simulink model "test_vacc_pkt_10_1_old"  (Simulink 7.2)
settings: Solver=ode45  StartTime=0.0  StopTime=5000  RelTol=1e-3
libraries: xbsIndex_r4 x248, xps_library x17, xbsReplacements_r4 x12, casper_library x5, casper_library_misc x2, casper_library_accumulators x1
(part 1 of 3)
settings Model: Creator=Jason Manley  LastModifiedBy=root
settings OptimizationCC: InitFltsAndDblsToZero=on
settings DebuggingCC: SaveWithParameterizedLinksMsg=none  SignalResolutionControl=TryResolveAllWithWarning  MultiTaskDSMMsg=warning  MultiTaskCondExecSysMsg=none  StrictBusMsg=None
settings RTWCC: IncludeERTFirstTime=on
settings GRTTargetCC: TargetFcnLib=ansi_tfl_tmw.mat

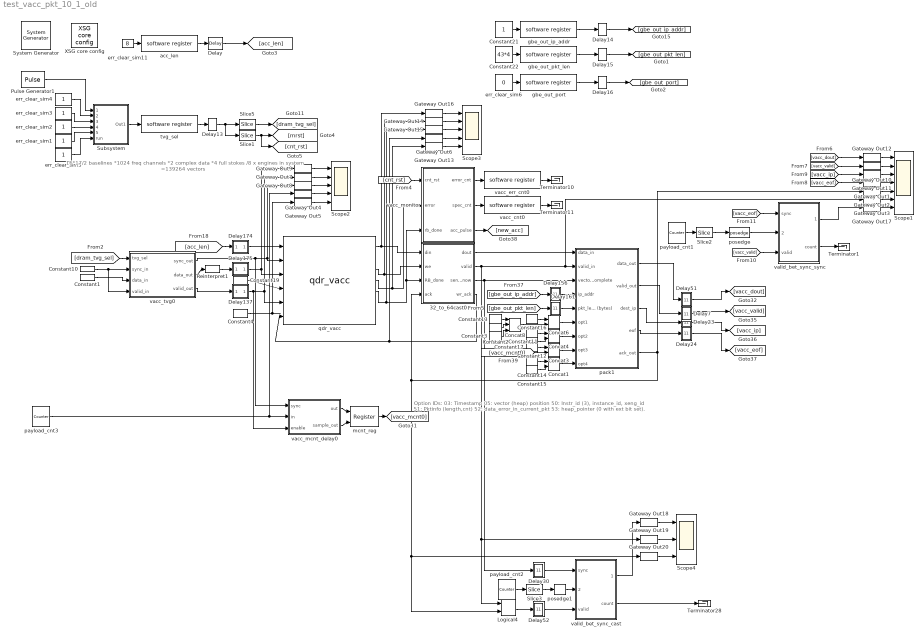
== system test_vacc_pkt_10_1_old ==
  note: 16*17/2 baselines
      | *1024 freq channels
      | *2 complex data
      | *4 full stokes
      | /8 x engines in system
      | =139264 vectors
  note: Option IDs:
      | 03: Timestamp
      | 05: vector (heap) position
      | 50: Instr_id (3), instance_id, xeng_id
      | 51: Pktinfo (length,cnt)
      | 52: data_error_in_current_pkt
      | 53: heap_pointer (0 with ext bit set).
  " System Generator" : xbsIndex_r4/ System Generator  Tag=genX  SystemSampleTime=-1  xilinxfamily=virtex5  part=xc5vlx110t  speed=-1  package=ff1136  synthesis_tool=XST  clock_wrapper=Clock Enables  directory=./test_vacc_pkt_10_1/sysgen  testbench=off  simulink_period=1  sysclk_period=5  dcm_input_clock_period=100  incr_netlist=off  trim_vbits=Everywhere in SubSystem  dbl_ovrd=According to Block Masks  core_generation=According to Block Masks  run_coregen=off  deprecated_control=off  eval_field=0  block_type=sysgen
      settings: block_version=10.1.3
  32_to_64cast0 : Subsystem
  Concat{1,3..4,6} (4 alike) : xbsIndex_r4/Concat  num_inputs=2  dbl_ovrd=off  block_type=concat
      settings: block_version=10.1.3
  Concat8 : xbsIndex_r4/Concat  num_inputs=3  dbl_ovrd=off  block_type=concat
      settings: block_version=10.1.3
  Constant1 : xbsIndex_r4/Constant  arith_type=Unsigned  const=0  n_bits=32  bin_pt=0  explicit_period=on  period=1  equ=P=C  opselect=C  inp2=PCIN>>17  opr=+  inp1=P  carry=CIN  dbl_ovrd=off  block_type=constant
  Constant10 : xbsIndex_r4/Constant  arith_type=Boolean  const=0  n_bits=1  bin_pt=0  explicit_period=on  period=1  equ=P=C  opselect=C  inp2=PCIN>>17  opr=+  inp1=P  carry=CIN  dbl_ovrd=off  block_type=constant
  Constant11 : xbsIndex_r4/Constant  arith_type=Unsigned  const=52  n_bits=16  bin_pt=0  explicit_period=on  period=1  equ=P=C  opselect=C  inp2=PCIN>>17  opr=+  inp1=P  carry=CIN  dbl_ovrd=off  block_type=constant
  Constant12 : xbsIndex_r4/Constant  arith_type=Unsigned  const=0  n_bits=48  bin_pt=0  explicit_period=on  period=1  equ=P=C  opselect=C  inp2=PCIN>>17  opr=+  inp1=P  carry=CIN  dbl_ovrd=off  block_type=constant
  Constant{2..3,13,17} (4 alike) : xbsIndex_r4/Constant  arith_type=Unsigned  const=3  n_bits=16  bin_pt=0  explicit_period=on  period=1  equ=P=C  opselect=C  inp2=PCIN>>17  opr=+  inp1=P  carry=CIN  dbl_ovrd=off  block_type=constant
  Constant14 : xbsIndex_r4/Constant  arith_type=Unsigned  const=53 + (1 * (2^15))  n_bits=16  bin_pt=0  explicit_period=on  period=1  equ=P=C  opselect=C  inp2=PCIN>>17  opr=+  inp1=P  carry=CIN  dbl_ovrd=off  block_type=constant
  Constant15 : xbsIndex_r4/Constant  arith_type=Unsigned  const=0  n_bits=48  bin_pt=0  explicit_period=on  period=1  equ=P=C  opselect=C  inp2=PCIN>>17  opr=+  inp1=P  carry=CIN  dbl_ovrd=off  block_type=constant
  Constant16 : xbsIndex_r4/Constant  arith_type=Unsigned  const=50  n_bits=16  bin_pt=0  explicit_period=on  period=1  equ=P=C  opselect=C  inp2=PCIN>>17  opr=+  inp1=P  carry=CIN  dbl_ovrd=off  block_type=constant
  Constant19 : xbsIndex_r4/Constant  arith_type=Unsigned  const=0  n_bits=4  bin_pt=0  explicit_period=on  period=1  equ=P=C  opselect=C  inp2=PCIN>>17  opr=+  inp1=P  carry=CIN  dbl_ovrd=off  block_type=constant
  Constant21 : Constant  OutDataType=sfix(16)  OutScaling=2^0
  Constant22 : Constant  Value=43*4  OutDataType=sfix(16)  OutScaling=2^0
  Constant4 : xbsIndex_r4/Constant  arith_type=Unsigned  const=0  n_bits=4  bin_pt=0  explicit_period=on  period=1  equ=P=C  opselect=C  inp2=PCIN>>17  opr=+  inp1=P  carry=CIN  dbl_ovrd=off  block_type=constant
  Delay : xbsIndex_r4/Delay  en=off  latency=1  dbl_ovrd=off  reg_retiming=on  block_type=delay
  Delay{13..16} (4 alike) : xbsIndex_r4/Delay  en=off  latency=2  dbl_ovrd=off  reg_retiming=on  block_type=delay
      settings: xl_area=[0, 0, 0, 0, 0, 0, 0]
  Delay137 : Subsystem  AncestorBlock=casper_library/Delays/pipeline  mask(pipeline){latency=2}
      mask help:
      | An explicitly laid-out delay line to avoid mapping to SRL16s
      | for use in pipelining to help achieve timing closure.
      mask init:
      | pipeline_init(gcb, 'latency', latency);
      mask Display:
      | port_label('input', 1, 'd');
      | port_label('output', 1, 'q');
      | disp(['Z^-', num2str(latency)]);
  Delay156 : Subsystem  AncestorBlock=casper_library/Delays/pipeline  mask(pipeline){latency=5}
      mask help:
      | An explicitly laid-out delay line to avoid mapping to SRL16s
      | for use in pipelining to help achieve timing closure.
      mask init:
      | pipeline_init(gcb, 'latency', latency);
      mask Display:
      | port_label('input', 1, 'd');
      | port_label('output', 1, 'q');
      | disp(['Z^-', num2str(latency)]);
  Delay161 : Subsystem  AncestorBlock=casper_library/Delays/pipeline  mask(pipeline){latency=1}
      mask help:
      | An explicitly laid-out delay line to avoid mapping to SRL16s
      | for use in pipelining to help achieve timing closure.
      mask init:
      | pipeline_init(gcb, 'latency', latency);
      mask Display:
      | port_label('input', 1, 'd');
      | port_label('output', 1, 'q');
      | disp(['Z^-', num2str(latency)]);
  Delay174 : Subsystem  AncestorBlock=casper_library/Delays/pipeline  mask(pipeline){latency=2}
      mask help:
      | An explicitly laid-out delay line to avoid mapping to SRL16s
      | for use in pipelining to help achieve timing closure.
      mask init:
      | pipeline_init(gcb, 'latency', latency);
      mask Display:
      | port_label('input', 1, 'd');
      | port_label('output', 1, 'q');
      | disp(['Z^-', num2str(latency)]);
  Delay175 : Subsystem  AncestorBlock=casper_library/Delays/pipeline  mask(pipeline){latency=2}
      mask help:
      | An explicitly laid-out delay line to avoid mapping to SRL16s
      | for use in pipelining to help achieve timing closure.
      mask init:
      | pipeline_init(gcb, 'latency', latency);
      mask Display:
      | port_label('input', 1, 'd');
      | port_label('output', 1, 'q');
      | disp(['Z^-', num2str(latency)]);
  Delay23 : Subsystem  AncestorBlock=casper_library/Delays/pipeline  mask(pipeline){latency=2}
      mask help:
      | An explicitly laid-out delay line to avoid mapping to SRL16s
      | for use in pipelining to help achieve timing closure.
      mask init:
      | pipeline_init(gcb, 'latency', latency);
      mask Display:
      | port_label('input', 1, 'd');
      | port_label('output', 1, 'q');
      | disp(['Z^-', num2str(latency)]);
  Delay24 : Subsystem  AncestorBlock=casper_library/Delays/pipeline  mask(pipeline){latency=2}
      mask help:
      | An explicitly laid-out delay line to avoid mapping to SRL16s
      | for use in pipelining to help achieve timing closure.
      mask init:
      | pipeline_init(gcb, 'latency', latency);
      mask Display:
      | port_label('input', 1, 'd');
      | port_label('output', 1, 'q');
      | disp(['Z^-', num2str(latency)]);
  Delay30 : Subsystem  AncestorBlock=casper_library/Delays/pipeline  mask(pipeline){latency=2}
      mask help:
      | An explicitly laid-out delay line to avoid mapping to SRL16s
      | for use in pipelining to help achieve timing closure.
      mask init:
      | pipeline_init(gcb, 'latency', latency);
      mask Display:
      | port_label('input', 1, 'd');
      | port_label('output', 1, 'q');
      | disp(['Z^-', num2str(latency)]);
  Delay51 : Subsystem  AncestorBlock=casper_library/Delays/pipeline  mask(pipeline){latency=2}
      mask help:
      | An explicitly laid-out delay line to avoid mapping to SRL16s
      | for use in pipelining to help achieve timing closure.
      mask init:
      | pipeline_init(gcb, 'latency', latency);
      mask Display:
      | port_label('input', 1, 'd');
      | port_label('output', 1, 'q');
      | disp(['Z^-', num2str(latency)]);
  Delay52 : Subsystem  AncestorBlock=casper_library/Delays/pipeline  mask(pipeline){latency=2}
      mask help:
      | An explicitly laid-out delay line to avoid mapping to SRL16s
      | for use in pipelining to help achieve timing closure.
      mask init:
      | pipeline_init(gcb, 'latency', latency);
      mask Display:
      | port_label('input', 1, 'd');
      | port_label('output', 1, 'q');
      | disp(['Z^-', num2str(latency)]);
  Delay7 : Subsystem  AncestorBlock=casper_library/Delays/pipeline  mask(pipeline){latency=2}
      mask help:
      | An explicitly laid-out delay line to avoid mapping to SRL16s
      | for use in pipelining to help achieve timing closure.
      mask init:
      | pipeline_init(gcb, 'latency', latency);
      mask Display:
      | port_label('input', 1, 'd');
      | port_label('output', 1, 'q');
      | disp(['Z^-', num2str(latency)]);
  Gateway Out{1..20} (20 alike) : xbsIndex_r4/Gateway Out  hdl_port=off  timing_constraint=None  locs_specified=off  LOCs={}  block_type=gatewayout
      settings: infoedit="Gateway out block.  Converts Xilinx fixed point inputs into ouputs of type Simulink integer, double, or fixed point.<P><P>Hardware notes:  In hardware these blocks become top level output ports or are discarded, depending on how they are configured."  xl_area=[0, 0, 0, 0, 0, 0, 0]  block_version=10.1.3
  Logical4 : xbsIndex_r4/Logical  logical_function=AND  inputs=2  en=off  latency=1  precision=Full  arith_type=Unsigned  n_bits=8  bin_pt=2  align_bp=on  dbl_ovrd=off  block_type=logical
      settings: xl_area=[0, 0, 0, 0, 0, 0, 0]
  Pulse Generator1 : DiscretePulseGenerator  Period=2*100*8  PhaseDelay=3
  Reinterpret1 : xbsIndex_r4/Reinterpret  force_arith_type=on  arith_type="Signed  (2's comp)"  force_bin_pt=on  bin_pt=0  block_type=reinterpret
      settings: infoedit="Changes signal type without altering the binary representation.   You can changed the signal between signed and unsigned, and relocate the binary point.<P><P>Hardware notes: In hardware this block costs nothing.<P><P>Example:  Suppose the input is 6 bits wide, signed, with 2 fractional bits, and the output is forced to unsigned with 0 fractional bits.  Then an input of -2.0 (1110.00 in binary 2's complement) becomes an output of 56 (111000 in binary)."  block_version=10.1.3
  Scope1 : Scope  NumInputPorts=7
      settings: YMin=0~0~0.95~0~0~0~493.05  YMax=1e+019~1~1.05~1~1~1~544.95  SaveName=ScopeData7
  Scope2 : Scope  NumInputPorts=5
      settings: YMin=0.95~0~-1~-5~-5  YMax=1.05~1~1~5~5  SaveName=ScopeData8
  Scope3 : Scope  NumInputPorts=5
      settings: YMin=0.95~0~-1~-5~-5  YMax=1.05~1~1~5~5  SaveName=ScopeData10
  Scope4 : Scope  NumInputPorts=3
      settings: YMin=61000~0~0  YMax=69500~1~1  SaveName=ScopeData11
  Slice1 : xbsIndex_r4/Slice  nbits=1  boolean_output=on  mode=Lower Bit Location + Width  bit1=0  base1=MSB of Input  bit0=31  base0=LSB of Input  dbl_ovrd=off  block_type=slice
      settings: infoedit="Extracts a given range of bits from each input sample and presents it at the output.  The output type is ordinarily unsigned with binary point at zero, but can be Boolean when the slice is one bit wide.<P><P>Hardware notes: In hardware this block costs nothing."  block_version=10.1.3
  Slice2 : xbsIndex_r4/Slice  nbits=1  boolean_output=on  mode=Upper Bit Location + Width  bit1=0  base1=MSB of Input  bit0=1  base0=LSB of Input  dbl_ovrd=off  block_type=slice
      settings: infoedit="Extracts a given range of bits from each input sample and presents it at the output.  The output type is ordinarily unsigned with binary point at zero, but can be Boolean when the slice is one bit wide.<P><P>Hardware notes: In hardware this block costs nothing."  block_version=10.1.3
  Slice3 : xbsIndex_r4/Slice  nbits=1  boolean_output=on  mode=Upper Bit Location + Width  bit1=0  base1=MSB of Input  bit0=1  base0=LSB of Input  dbl_ovrd=off  block_type=slice
      settings: infoedit="Extracts a given range of bits from each input sample and presents it at the output.  The output type is ordinarily unsigned with binary point at zero, but can be Boolean when the slice is one bit wide.<P><P>Hardware notes: In hardware this block costs nothing."  block_version=10.1.3
  Slice5 : xbsIndex_r4/Slice  nbits=6  boolean_output=off  mode=Lower Bit Location + Width  bit1=0  base1=MSB of Input  bit0=9  base0=LSB of Input  dbl_ovrd=off  block_type=slice
      settings: infoedit="Extracts a given range of bits from each input sample and presents it at the output.  The output type is ordinarily unsigned with binary point at zero, but can be Boolean when the slice is one bit wide.<P><P>Hardware notes: In hardware this block costs nothing."  block_version=10.1.3
  Subsystem : Subsystem
  Terminator{1,10..11,28} (4 alike) : Terminator
  XSG core config : xps_library/XSG core config  Tag=xps:xsg  SystemSampleTime=-1  hw_sys=iBOB  ibob_linux=off  clk_src=sys_clk  iBOB_clk_src=sys_clk  BEE2_ctrl_clk_src=sys_clk  BEE2_usr_clk_src=sys_clk  ROACH_clk_src=arb_clk  CORR_clk_src=sys_clk  gpio_clk_io_group=iBOB:sma  gpio_clk_bit_index=0  clk_rate=100  sample_period=1  synthesis_tool=XST  mpc_type=powerpc405
  acc_len : xps_library/software register  Tag=xps:sw_reg  SystemSampleTime=-1  io_dir=From Processor  arith_type=Unsigned  bitwidth=32  bin_pt=0  sample_period=1  gw_name=test_vacc_pkt_10_1_acc_len_user_data_out
      link override qdr_vacc_tvg_sel_user_data_out: arith_type=Unsigned  n_bits=32  bin_pt=0  period=1
      link override test_d_v_p_10_1_new_packet_format_acc_len_user_data_out: arith_type=Unsigned  n_bits=32  bin_pt=0  period=1
      link override test_qdr_vacc_acc_len_user_data_out: arith_type=Unsigned  n_bits=32  bin_pt=0  period=1
      link override test_qdr_vacc_tvg_sel_user_data_out: arith_type=Unsigned  n_bits=32  bin_pt=0  period=1
      link override test_vacc_10_1_new_pkt_form_acc_len_user_data_out: arith_type=Unsigned  n_bits=32  bin_pt=0  period=1
      link override test_vacc_pkt_10_1_acc_len_user_data_out: arith_type=Unsigned  n_bits=32  bin_pt=0  period=1
  err_clear_sim{1..5} (5 alike) : Constant  OutDataType=sfix(16)  OutScaling=2^0
  err_clear_sim11 : Constant  Value=8  OutDataType=sfix(16)  OutScaling=2^0
  err_clear_sim6 : Constant  Value=0  OutDataType=sfix(16)  OutScaling=2^0
  gbe_out_ip_addr : xps_library/software register  Tag=xps:sw_reg  SystemSampleTime=-1  io_dir=From Processor  arith_type=Unsigned  bitwidth=32  bin_pt=0  sample_period=1  gw_name=test_vacc_pkt_10_1_gbe_out_ip_addr_user_data_out
      link override test_d_v_p_10_1_new_packet_format_gbe_out_ip_addr_user_data_out: arith_type=Unsigned  n_bits=32  bin_pt=0  period=1
      link override test_d_v_p_10_1_new_packet_format_out_ip_addr_user_data_out: arith_type=Unsigned  n_bits=32  bin_pt=0  period=1
      link override test_vacc_10_1_new_pkt_form_gbe_out_ip_addr_user_data_out: arith_type=Unsigned  n_bits=32  bin_pt=0  period=1
      link override test_vacc_pkt_10_1_gbe_out_ip_addr_user_data_out: arith_type=Unsigned  n_bits=32  bin_pt=0  period=1
  gbe_out_pkt_len : xps_library/software register  Tag=xps:sw_reg  SystemSampleTime=-1  io_dir=From Processor  arith_type=Unsigned  bitwidth=32  bin_pt=0  sample_period=1  gw_name=test_vacc_pkt_10_1_gbe_out_pkt_len_user_data_out
      link override test_d_v_p_10_1_new_packet_format_gbe_out_pkt_len_user_data_out: arith_type=Unsigned  n_bits=32  bin_pt=0  period=1
      link override test_d_v_p_10_1_new_packet_format_pkt_len_user_data_out: arith_type=Unsigned  n_bits=32  bin_pt=0  period=1
      link override test_vacc_10_1_new_pkt_form_gbe_out_pkt_len_user_data_out: arith_type=Unsigned  n_bits=32  bin_pt=0  period=1
      link override test_vacc_pkt_10_1_gbe_out_pkt_len_user_data_out: arith_type=Unsigned  n_bits=32  bin_pt=0  period=1
  gbe_out_port : xps_library/software register  Tag=xps:sw_reg  SystemSampleTime=-1  io_dir=From Processor  arith_type=Unsigned  bitwidth=32  bin_pt=0  sample_period=1  gw_name=test_vacc_pkt_10_1_gbe_out_port_user_data_out
      link override test_d_v_p_10_1_new_packet_format_gbe_out_port_user_data_out: arith_type=Unsigned  n_bits=32  bin_pt=0  period=1
      link override test_vacc_10_1_new_pkt_form_gbe_out_port_user_data_out: arith_type=Unsigned  n_bits=32  bin_pt=0  period=1
      link override test_vacc_pkt_10_1_gbe_out_port_user_data_out: arith_type=Unsigned  n_bits=32  bin_pt=0  period=1
  mcnt_reg : xbsIndex_r4/Register  init=0  rst=off  en=on  dbl_ovrd=off  block_type=register
  pack1 : Subsystem  mask(pkt_pack_mask){vector_len=100, magic_id=hex2dec('4b52'), ver_id=3}
      mask prompts: vector_len "vector length"; magic_id "Magic Identifier"; ver_id "Version Identifier"
      mask help:
      | This block generates packets from a datastream.
      |
      | Packets are created with a fixed header followed by a user-specified number of 64-bit options.
      |
      | Requires a 64-bit data stream.
      |
      | See the documentation for further details.
      mask init:
      | vector_bits = ceil(log2(vector_len));
  payload_cnt1 : xbsIndex_r4/Counter  cnt_type=Free Running  cnt_to=0  operation=Up  start_count=0  cnt_by_val=1  arith_type=Unsigned  n_bits=12  bin_pt=0  load_pin=off  rst=off  en=off  explicit_period=on  period=1  dbl_ovrd=off  use_behavioral_HDL=off  implementation=Fabric  use_rpm=on  block_type=counter
      settings: xl_area=[0, 0, 0, 0, 0, 0, 0]
  payload_cnt2 : xbsIndex_r4/Counter  cnt_type=Free Running  cnt_to=0  operation=Up  start_count=0  cnt_by_val=1  arith_type=Unsigned  n_bits=19  bin_pt=0  load_pin=off  rst=off  en=off  explicit_period=on  period=1  dbl_ovrd=off  use_behavioral_HDL=off  implementation=Fabric  use_rpm=on  block_type=counter
      settings: xl_area=[0, 0, 0, 0, 0, 0, 0]
  payload_cnt3 : xbsIndex_r4/Counter  cnt_type=Free Running  cnt_to=0  operation=Up  start_count=0  cnt_by_val=1  arith_type=Unsigned  n_bits=48  bin_pt=0  load_pin=off  rst=off  en=off  explicit_period=on  period=1  dbl_ovrd=off  use_behavioral_HDL=off  implementation=Fabric  use_rpm=on  block_type=counter
      settings: xl_area=[0, 0, 0, 0, 0, 0, 0]
  posedge : casper_library_misc/posedge  Tag=Rising Edge Detector  SystemSampleTime=-1
  posedge1 : casper_library_misc/posedge  Tag=Rising Edge Detector  SystemSampleTime=-1
  qdr_vacc : casper_library_accumulators/qdr_vacc  SystemSampleTime=-1  vector_len=100
      settings: AttributesFormatString=Vector Length: 100
  tvg_sel : xps_library/software register  Tag=xps:sw_reg  SystemSampleTime=-1  io_dir=From Processor  arith_type=Unsigned  bitwidth=32  bin_pt=0  sample_period=1  gw_name=test_vacc_pkt_10_1_tvg_sel_user_data_out
      link override test_d_v_p_10_1_new_packet_format_tvg_sel_user_data_out: arith_type=Unsigned  n_bits=32  bin_pt=0  period=1
      link override test_vacc_10_1_new_pkt_form_tvg_sel_user_data_out: arith_type=Unsigned  n_bits=32  bin_pt=0  period=1
      link override test_vacc_pkt_10_1_tvg_sel_user_data_out: arith_type=Unsigned  n_bits=32  bin_pt=0  period=1
  vacc_cnt0 : xps_library/software register  Tag=xps:sw_reg  SystemSampleTime=-1  io_dir=To Processor  arith_type=Unsigned  bitwidth=32  bin_pt=0  sample_period=1  gw_name=test_vacc_pkt_10_1_vacc_cnt0_user_data_in
      link override convert: arith_type=Unsigned  n_bits=32  bin_pt=0
  vacc_err_cnt0 : xps_library/software register  Tag=xps:sw_reg  SystemSampleTime=-1  io_dir=To Processor  arith_type=Unsigned  bitwidth=32  bin_pt=0  sample_period=1  gw_name=test_vacc_pkt_10_1_vacc_err_cnt0_user_data_in
      link override convert: arith_type=Unsigned  n_bits=32  bin_pt=0
  vacc_mcnt_delay0 : Subsystem  mask(sample_and_hold){period=16*17/2*1024*2*4/8}
      mask prompts: period "Sample period (clocks)"
      mask help: This block will sample an input signal at a user specified rate and hold the value on the output.
  vacc_monitor : Subsystem
  vacc_tvg0 : Subsystem  AncestorBlock=casper_library/Accumulators/vacc_tvg  mask{len=100}
      mask prompts: len "Number of Vectors"
      mask init:
      | fmtstr = sprintf('Vector Length: %d', len);
      | set_param(gcb, 'AttributesFormatString', fmtstr);
      settings: AttributesFormatString=Vector Length: 100
  valid_bet_sync_cast : Subsystem
  valid_bet_sync_sync : Subsystem
  wires:
  tvg_sel/1 -> Delay13/1
  Slice5/1 -> [dram_tvg_sel]
  err_clear_sim1/1 -> Subsystem/5(data_sel)
  err_clear_sim2/1 -> Subsystem/4(valid_sel)
  err_clear_sim3/1 -> Subsystem/3(inj_vector)
  err_clear_sim4/1 -> Subsystem/2(inj_counter)
  Subsystem/1(Out1) -> tvg_sel/1
  Pulse Generator1/1 -> Subsystem/1(new_acc)
  err_clear_sim5/1 -> Subsystem/6(run)
  Constant22/1 -> gbe_out_pkt_len/1
  Constant21/1 -> gbe_out_ip_addr/1
  gbe_out_ip_addr/1 -> Delay14/1
  gbe_out_pkt_len/1 -> Delay15/1
  Slice1/1 -> [mrst], [cnt_rst]
  acc_len/1 -> Delay/1
  err_clear_sim11/1 -> acc_len/1
  err_clear_sim6/1 -> gbe_out_port/1
  gbe_out_port/1 -> Delay16/1
  Delay13/1 -> Slice5/1, Slice1/1
  Delay14/1 -> [gbe_out_ip_addr]
  Delay15/1 -> [gbe_out_pkt_len]
  Delay16/1 -> [gbe_out_port]
  qdr_vacc/1 -> 32_to_64cast0/1(din), Gateway Out16/1
  qdr_vacc/3 -> 32_to_64cast0/2(we), Gateway Out14/1
  qdr_vacc/5 -> 32_to_64cast0/3(RB_done), vacc_monitor/3(rb_done), Gateway Out15/1
  [acc_len] -> Delay174/1(d)
  Delay174/1(q) -> qdr_vacc/1
  Delay175/1(q) -> Gateway Out9/1, qdr_vacc/3
  Delay137/1(q) -> vacc_mcnt_delay0/3(enable), Gateway Out7/1, qdr_vacc/5
  [gbe_out_ip_addr] -> Delay156/1(d)
  [gbe_out_pkt_len] -> Delay161/1(d)
  Delay156/1(q) -> pack1/4(ip_addr)
  Delay161/1(q) -> pack1/5(pkt_len (bytes))
  pack1/4(eof) -> Delay24/1(d)
  pack1/5(ack_out) -> Gateway Out2/1, 32_to_64cast0/4(ack), Logical4/2, Gateway Out20/1
  pack1/1(data_out) -> Delay51/1(d)
  pack1/2(valid_out) -> Delay7/1(d)
  32_to_64cast0/1(dout) -> pack1/1(data_in)
  32_to_64cast0/2(valid) -> pack1/2(valid_in), Gateway Out3/1, Logical4/1, Gateway Out19/1
  32_to_64cast0/3(send_now) -> pack1/3(vector_complete), Delay30/1(d)
  32_to_64cast0/4(wr_ack) -> Gateway Out6/1, qdr_vacc/6
  pack1/3(dest_ip) -> Delay23/1(d)
  Constant4/1 -> Gateway Out5/1
  Constant19/1 -> qdr_vacc/4
  Delay51/1(q) -> [vacc_dout]
  Delay7/1(q) -> [vacc_valid]
  Delay23/1(q) -> [vacc_ip]
  Delay24/1(q) -> [vacc_eof]
  vacc_tvg0/1(sync_out) -> vacc_mcnt_delay0/1(sync), Gateway Out8/1, qdr_vacc/2
  vacc_tvg0/2(data_out) -> Reinterpret1/1
  vacc_tvg0/3(valid_out) -> Delay137/1(d)
  vacc_mcnt_delay0/1(out) -> mcnt_reg/1
  vacc_mcnt_delay0/2(sample_out) -> mcnt_reg/2
  Constant17/1 -> Concat3/1
  [vacc_mcnt0] -> Concat3/2
  mcnt_reg/1 -> [vacc_mcnt0]
  Concat3/1 -> pack1/8(opt3)
  Concat6/1 -> pack1/6(opt1)
  Constant16/1 -> Concat6/1
  Concat4/1 -> pack1/7(opt2)
  Concat1/1 -> pack1/9(opt4)
  vacc_cnt0/1 -> Terminator11/1
  vacc_monitor/2(spec_cnt) -> vacc_cnt0/1
  Reinterpret1/1 -> Delay175/1(d)
  vacc_err_cnt0/1 -> Terminator10/1
  vacc_monitor/1(error_cnt) -> vacc_err_cnt0/1
  qdr_vacc/4 -> vacc_monitor/2(error), Gateway Out13/1
  vacc_monitor/3(acc_pulse) -> [new_acc]
  [cnt_rst] -> vacc_monitor/1(cnt_rst)
  Concat8/1 -> Concat6/2
  Constant13/1 -> Concat8/1
  Constant2/1 -> Concat8/2
  Constant3/1 -> Concat8/3
  Constant14/1 -> Concat1/1
  Constant15/1 -> Concat1/2
  Constant11/1 -> Concat4/1
  Constant12/1 -> Concat4/2
  Delay/1 -> [acc_len]
  [dram_tvg_sel] -> vacc_tvg0/1(tvg_sel)
  Constant10/1 -> vacc_tvg0/2(sync_in), vacc_tvg0/4(valid_in)
  Constant1/1 -> vacc_tvg0/3(data_in)
  payload_cnt3/1 -> vacc_mcnt_delay0/2(in), Gateway Out4/1
  Gateway Out5/1 -> Scope2/5
  Gateway Out4/1 -> Scope2/4
  Gateway Out9/1 -> Scope2/1
  Gateway Out7/1 -> Scope2/2
  Gateway Out8/1 -> Scope2/3
  Gateway Out3/1 -> Scope1/6
  Gateway Out2/1 -> Scope1/5
  Gateway Out1/1 -> Scope1/4
  Gateway Out12/1 -> Scope1/1
  Gateway Out10/1 -> Scope1/2
  Gateway Out11/1 -> Scope1/3
  [vacc_dout] -> Gateway Out12/1
  [vacc_valid] -> Gateway Out10/1
  [vacc_ip] -> Gateway Out11/1
  [vacc_eof] -> Gateway Out1/1
  Gateway Out13/1 -> Scope3/5
  Gateway Out6/1 -> Scope3/4
  Gateway Out16/1 -> Scope3/1
  Gateway Out14/1 -> Scope3/2
  Gateway Out15/1 -> Scope3/3
  valid_bet_sync_sync/2(count) -> Terminator1/1
  [vacc_valid] -> valid_bet_sync_sync/3(valid)
  [vacc_eof] -> valid_bet_sync_sync/1(sync)
  payload_cnt1/1 -> Slice2/1
  Slice2/1 -> posedge/1
  Gateway Out17/1 -> Scope1/7
  posedge/1 -> valid_bet_sync_sync/2(rst_max)
  Logical4/1 -> Delay52/1(d)
  valid_bet_sync_cast/2(count) -> Terminator28/1
  valid_bet_sync_cast/1(max_count) -> Gateway Out18/1
  Delay30/1(q) -> valid_bet_sync_cast/1(sync)
  Slice3/1 -> posedge1/1
  Delay52/1(q) -> valid_bet_sync_cast/3(valid)
  Gateway Out18/1 -> Scope4/1
  Gateway Out19/1 -> Scope4/2
  Gateway Out20/1 -> Scope4/3
  payload_cnt2/1 -> Slice3/1
  posedge1/1 -> valid_bet_sync_cast/2(rst_max)
  valid_bet_sync_sync/1(max_count) -> Gateway Out17/1

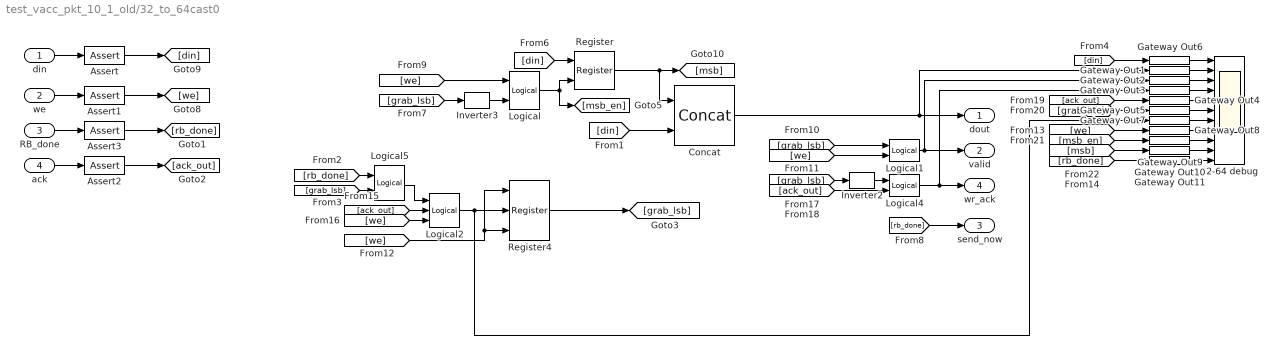
== system test_vacc_pkt_10_1_old/32_to_64cast0 ==
  din : Inport  OutDataType=sfix(16)  OutScaling=2^0
  we : Inport  Port=2  OutDataType=sfix(16)  OutScaling=2^0
  RB_done : Inport  Port=3  OutDataType=sfix(16)  OutScaling=2^0
  ack : Inport  Port=4  OutDataType=sfix(16)  OutScaling=2^0
  32-64 debug : Scope  NumInputPorts=11
      settings: YMin=-1~0~0~0~-5~-5~-5~-5~-5~-5~-5  YMax=1~150~1~1~5~5~5~5~5~5~5  SaveName=ScopeData5
  Assert : xbsIndex_r4/Assert  assert_type=on  type_source=Explicitly  arith_type=Unsigned  n_bits=32  bin_pt=0  assert_rate=off  rate_source=Explicitly  period=1  output_port=on  block_type=assert
      settings: infoedit=Asserts a user-defined sample rate and/or type on a signal.<P><P>Hardware notes: In hardware this block costs nothing.  block_version=10.1.3
  Assert1 : xbsIndex_r4/Assert  assert_type=on  type_source=Explicitly  arith_type=Boolean  n_bits=32  bin_pt=0  assert_rate=off  rate_source=Explicitly  period=1  output_port=on  block_type=assert
      settings: infoedit=Asserts a user-defined sample rate and/or type on a signal.<P><P>Hardware notes: In hardware this block costs nothing.  block_version=10.1.3
  Assert2 : xbsIndex_r4/Assert  assert_type=on  type_source=Explicitly  arith_type=Boolean  n_bits=32  bin_pt=0  assert_rate=off  rate_source=Explicitly  period=1  output_port=on  block_type=assert
      settings: infoedit=Asserts a user-defined sample rate and/or type on a signal.<P><P>Hardware notes: In hardware this block costs nothing.  block_version=10.1.3
  Assert3 : xbsIndex_r4/Assert  assert_type=on  type_source=Explicitly  arith_type=Boolean  n_bits=32  bin_pt=0  assert_rate=off  rate_source=Explicitly  period=1  output_port=on  block_type=assert
      settings: infoedit=Asserts a user-defined sample rate and/or type on a signal.<P><P>Hardware notes: In hardware this block costs nothing.  block_version=10.1.3
  Concat : xbsIndex_r4/Concat  num_inputs=2  dbl_ovrd=off  block_type=concat
      settings: block_version=10.1.3
  Gateway Out{1..11} (11 alike) : xbsIndex_r4/Gateway Out  hdl_port=off  timing_constraint=None  locs_specified=off  LOCs={}  block_type=gatewayout
      settings: infoedit="Gateway out block.  Converts Xilinx fixed point inputs into ouputs of type Simulink integer, double, or fixed point.<P><P>Hardware notes:  In hardware these blocks become top level output ports or are discarded, depending on how they are configured."  xl_area=[0, 0, 0, 0, 0, 0, 0]  block_version=10.1.3
  Inverter2 : xbsIndex_r4/Inverter  en=off  latency=0  dbl_ovrd=off  block_type=inv
  Inverter3 : xbsIndex_r4/Inverter  en=off  latency=0  dbl_ovrd=off  block_type=inv
  Logical : xbsIndex_r4/Logical  logical_function=AND  inputs=2  en=off  latency=0  precision=Full  arith_type=Unsigned  n_bits=16  bin_pt=0  align_bp=on  dbl_ovrd=off  block_type=logical
  Logical1 : xbsIndex_r4/Logical  logical_function=AND  inputs=2  en=off  latency=0  precision=Full  arith_type=Unsigned  n_bits=16  bin_pt=0  align_bp=on  dbl_ovrd=off  block_type=logical
  Logical2 : xbsIndex_r4/Logical  logical_function=AND  inputs=3  en=off  latency=0  precision=Full  arith_type=Unsigned  n_bits=16  bin_pt=0  align_bp=on  dbl_ovrd=off  block_type=logical
  Logical4 : xbsIndex_r4/Logical  logical_function=OR  inputs=2  en=off  latency=0  precision=Full  arith_type=Unsigned  n_bits=16  bin_pt=0  align_bp=on  dbl_ovrd=off  block_type=logical
  Logical5 : xbsIndex_r4/Logical  logical_function=OR  inputs=2  en=off  latency=0  precision=Full  arith_type=Unsigned  n_bits=16  bin_pt=0  align_bp=on  dbl_ovrd=off  block_type=logical
  Register : xbsIndex_r4/Register  init=0  rst=off  en=on  dbl_ovrd=off  block_type=register
  Register4 : xbsIndex_r4/Register  init=0  rst=on  en=on  dbl_ovrd=off  block_type=register
  dout : Outport  OutDataType=sfix(16)  OutScaling=2^0
  valid : Outport  Port=2  OutDataType=sfix(16)  OutScaling=2^0
  send_now : Outport  Port=3  OutDataType=sfix(16)  OutScaling=2^0
  wr_ack : Outport  Port=4  OutDataType=sfix(16)  OutScaling=2^0
  wires:
  din/1 -> Assert/1
  ack/1 -> Assert2/1
  we/1 -> Assert1/1
  Assert/1 -> [din]
  Assert1/1 -> [we]
  Assert2/1 -> [ack_out]
  [din] -> Register/1
  Register/1 -> Concat/1, [msb]
  [din] -> Concat/2
  Logical4/1 -> wr_ack/1, Gateway Out3/1
  Logical1/1 -> valid/1, Gateway Out2/1
  Logical/1 -> Register/2, [msb_en]
  RB_done/1 -> Assert3/1
  Assert3/1 -> [rb_done]
  [rb_done] -> send_now/1
  Concat/1 -> dout/1, Gateway Out1/1
  Register4/1 -> [grab_lsb]
  [grab_lsb] -> Inverter3/1
  [we] -> Logical/1
  [grab_lsb] -> Inverter2/1
  [ack_out] -> Logical4/2
  Gateway Out6/1 -> 32-64 debug/1
  Gateway Out1/1 -> 32-64 debug/2
  Gateway Out2/1 -> 32-64 debug/3
  Gateway Out3/1 -> 32-64 debug/4
  [din] -> Gateway Out6/1
  [ack_out] -> Gateway Out4/1
  [grab_lsb] -> Gateway Out5/1
  Gateway Out4/1 -> 32-64 debug/5
  Gateway Out5/1 -> 32-64 debug/6
  Gateway Out7/1 -> 32-64 debug/7
  Gateway Out8/1 -> 32-64 debug/8
  Gateway Out9/1 -> 32-64 debug/9
  Gateway Out10/1 -> 32-64 debug/10
  [we] -> Gateway Out8/1
  [msb_en] -> Gateway Out9/1
  [msb] -> Gateway Out10/1
  [we] -> Logical1/2
  [grab_lsb] -> Logical1/1
  Inverter2/1 -> Logical4/1
  Inverter3/1 -> Logical/2
  [rb_done] -> Gateway Out11/1
  Gateway Out11/1 -> 32-64 debug/11
  Logical5/1 -> Logical2/1
  [ack_out] -> Logical2/2
  [we] -> Logical2/3
  [rb_done] -> Logical5/1
  Logical2/1 -> Register4/2, Gateway Out7/1
  [grab_lsb] -> Logical5/2
  [we] -> Register4/3, Register4/1

== system test_vacc_pkt_10_1_old/Delay137 ==
  d : Inport
  Register0 : xbsIndex_r4/Register  init=0  rst=off  en=off  dbl_ovrd=off  block_type=register
  Register1 : xbsIndex_r4/Register  init=0  rst=off  en=off  dbl_ovrd=off  block_type=register
  q : Outport
  wires:
  Register0/1 -> Register1/1
  d/1 -> Register0/1
  Register1/1 -> q/1

== system test_vacc_pkt_10_1_old/Delay156 ==
  d : Inport
  Register{0..4} (5 alike) : xbsIndex_r4/Register  init=0  rst=off  en=off  dbl_ovrd=off  block_type=register
  q : Outport
  wires:
  Register0/1 -> Register1/1
  Register1/1 -> Register2/1
  Register2/1 -> Register3/1
  Register3/1 -> Register4/1
  d/1 -> Register0/1
  Register4/1 -> q/1

== system test_vacc_pkt_10_1_old/Delay161 ==
  d : Inport
  Register0 : xbsIndex_r4/Register  init=0  rst=off  en=off  dbl_ovrd=off  block_type=register
  q : Outport
  wires:
  d/1 -> Register0/1
  Register0/1 -> q/1

== system test_vacc_pkt_10_1_old/Delay174 ==
  d : Inport
  Register0 : xbsIndex_r4/Register  init=0  rst=off  en=off  dbl_ovrd=off  block_type=register
  Register1 : xbsIndex_r4/Register  init=0  rst=off  en=off  dbl_ovrd=off  block_type=register
  q : Outport
  wires:
  Register0/1 -> Register1/1
  d/1 -> Register0/1
  Register1/1 -> q/1

== system test_vacc_pkt_10_1_old/Delay175 ==
  d : Inport
  Register0 : xbsIndex_r4/Register  init=0  rst=off  en=off  dbl_ovrd=off  block_type=register
  Register1 : xbsIndex_r4/Register  init=0  rst=off  en=off  dbl_ovrd=off  block_type=register
  q : Outport
  wires:
  Register0/1 -> Register1/1
  d/1 -> Register0/1
  Register1/1 -> q/1

== system test_vacc_pkt_10_1_old/Delay23 ==
  d : Inport
  Register0 : xbsIndex_r4/Register  init=0  rst=off  en=off  dbl_ovrd=off  block_type=register
  Register1 : xbsIndex_r4/Register  init=0  rst=off  en=off  dbl_ovrd=off  block_type=register
  q : Outport
  wires:
  Register0/1 -> Register1/1
  d/1 -> Register0/1
  Register1/1 -> q/1

== system test_vacc_pkt_10_1_old/Delay24 ==
  d : Inport
  Register0 : xbsIndex_r4/Register  init=0  rst=off  en=off  dbl_ovrd=off  block_type=register
  Register1 : xbsIndex_r4/Register  init=0  rst=off  en=off  dbl_ovrd=off  block_type=register
  q : Outport
  wires:
  Register0/1 -> Register1/1
  d/1 -> Register0/1
  Register1/1 -> q/1

== system test_vacc_pkt_10_1_old/Delay30 ==
  d : Inport
  Register0 : xbsIndex_r4/Register  init=0  rst=off  en=off  dbl_ovrd=off  block_type=register
  Register1 : xbsIndex_r4/Register  init=0  rst=off  en=off  dbl_ovrd=off  block_type=register
  q : Outport
  wires:
  Register0/1 -> Register1/1
  d/1 -> Register0/1
  Register1/1 -> q/1

== system test_vacc_pkt_10_1_old/Delay51 ==
  d : Inport
  Register0 : xbsIndex_r4/Register  init=0  rst=off  en=off  dbl_ovrd=off  block_type=register
  Register1 : xbsIndex_r4/Register  init=0  rst=off  en=off  dbl_ovrd=off  block_type=register
  q : Outport
  wires:
  Register0/1 -> Register1/1
  d/1 -> Register0/1
  Register1/1 -> q/1

== system test_vacc_pkt_10_1_old/Delay52 ==
  d : Inport
  Register0 : xbsIndex_r4/Register  init=0  rst=off  en=off  dbl_ovrd=off  block_type=register
  Register1 : xbsIndex_r4/Register  init=0  rst=off  en=off  dbl_ovrd=off  block_type=register
  q : Outport
  wires:
  Register0/1 -> Register1/1
  d/1 -> Register0/1
  Register1/1 -> q/1

== system test_vacc_pkt_10_1_old/Delay7 ==
  d : Inport
  Register0 : xbsIndex_r4/Register  init=0  rst=off  en=off  dbl_ovrd=off  block_type=register
  Register1 : xbsIndex_r4/Register  init=0  rst=off  en=off  dbl_ovrd=off  block_type=register
  q : Outport
  wires:
  Register0/1 -> Register1/1
  d/1 -> Register0/1
  Register1/1 -> q/1

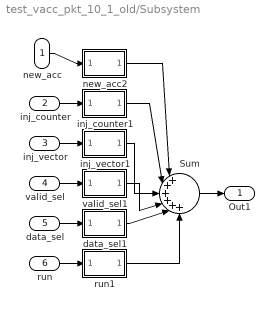
== system test_vacc_pkt_10_1_old/Subsystem ==
  new_acc : Inport  OutDataType=sfix(16)  OutScaling=2^0
  inj_counter : Inport  Port=2  OutDataType=sfix(16)  OutScaling=2^0
  inj_vector : Inport  Port=3  OutDataType=sfix(16)  OutScaling=2^0
  valid_sel : Inport  Port=4  OutDataType=sfix(16)  OutScaling=2^0
  data_sel : Inport  Port=5  OutDataType=sfix(16)  OutScaling=2^0
  run : Inport  Port=6  OutDataType=sfix(16)  OutScaling=2^0
  Sum : Sum  Inputs=|++++++  OutDataType=sfix(16)  OutScaling=2^0
  data_sel1 : Subsystem  mask{bit_pos=10}
      mask prompts: bit_pos "bit position"
  inj_counter1 : Subsystem  mask{bit_pos=13}
      mask prompts: bit_pos "bit position"
  inj_vector1 : Subsystem  mask{bit_pos=12}
      mask prompts: bit_pos "bit position"
  new_acc2 : Subsystem  mask{bit_pos=14}
      mask prompts: bit_pos "bit position"
  run1 : Subsystem  mask{bit_pos=9}
      mask prompts: bit_pos "bit position"
  valid_sel1 : Subsystem  mask{bit_pos=11}
      mask prompts: bit_pos "bit position"
  Out1 : Outport  OutDataType=sfix(16)  OutScaling=2^0
  wires:
  new_acc2/1(Out1) -> Sum/1
  inj_counter1/1(Out1) -> Sum/2
  inj_vector1/1(Out1) -> Sum/3
  valid_sel1/1(Out1) -> Sum/4
  data_sel1/1(Out1) -> Sum/5
  run1/1(Out1) -> Sum/6
  new_acc/1 -> new_acc2/1(In1)
  inj_counter/1 -> inj_counter1/1(In1)
  inj_vector/1 -> inj_vector1/1(In1)
  valid_sel/1 -> valid_sel1/1(In1)
  Sum/1 -> Out1/1
  data_sel/1 -> data_sel1/1(In1)
  run/1 -> run1/1(In1)

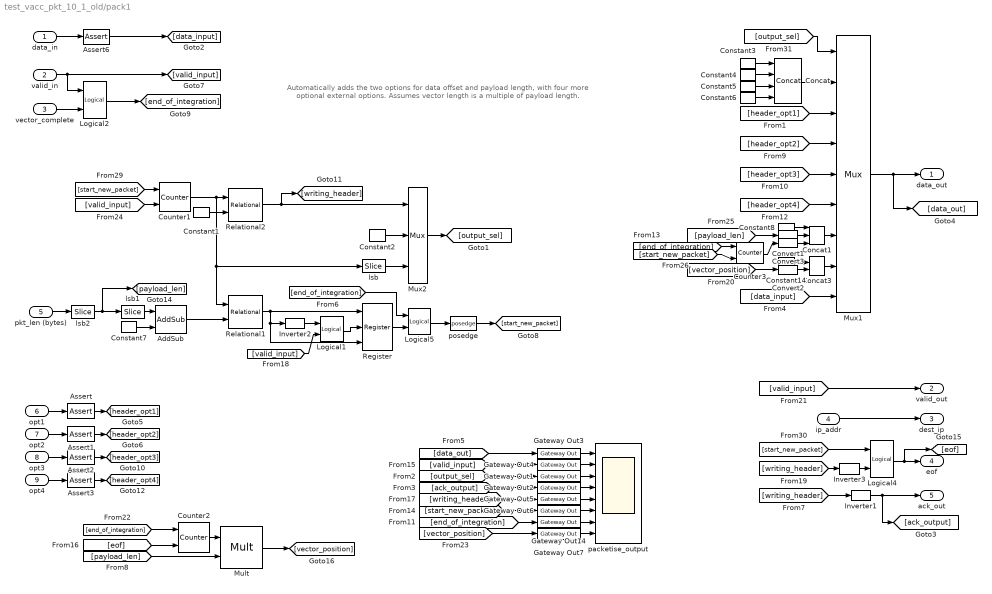
== system test_vacc_pkt_10_1_old/pack1 ==
  note: Automatically adds the two options for data offset and
      | payload length, with four more optional external options.
      | Assumes vector length is a multiple of payload length.
  data_in : Inport  OutDataType=sfix(16)  OutScaling=2^0
  valid_in : Inport  Port=2  OutDataType=sfix(16)  OutScaling=2^0
  vector_complete : Inport  Port=3  OutDataType=sfix(16)  OutScaling=2^0
  ip_addr : Inport  Port=4  OutDataType=sfix(16)  OutScaling=2^0
  pkt_len (bytes) : Inport  Port=5  OutDataType=sfix(16)  OutScaling=2^0
  opt1 : Inport  Port=6  OutDataType=sfix(16)  OutScaling=2^0
  opt2 : Inport  Port=7  OutDataType=sfix(16)  OutScaling=2^0
  opt3 : Inport  Port=8  OutDataType=sfix(16)  OutScaling=2^0
  opt4 : Inport  Port=9  OutDataType=sfix(16)  OutScaling=2^0
  AddSub : xbsIndex_r4/AddSub  mode=Addition  use_carryin=off  use_carryout=off  en=off  latency=0  precision=Full  arith_type=Unsigned  n_bits=16  bin_pt=14  quantization=Truncate  overflow=Wrap  dbl_ovrd=off  use_behavioral_HDL=off  pipelined=off  use_rpm=on  hw_selection=Fabric  block_type=addsub
      settings: block_version=10.1.3
  Assert{,1..3,6} (5 alike) : xbsIndex_r4/Assert  assert_type=on  type_source=Explicitly  arith_type=Unsigned  n_bits=64  bin_pt=0  assert_rate=off  rate_source=Explicitly  period=1  output_port=on  block_type=assert
      settings: infoedit=Asserts a user-defined sample rate and/or type on a signal.<P><P>Hardware notes: In hardware this block costs nothing.  block_version=10.1.3
  Concat : xbsIndex_r4/Concat  num_inputs=4  dbl_ovrd=off  block_type=concat
      settings: block_version=10.1.3
  Concat1 : xbsIndex_r4/Concat  num_inputs=3  dbl_ovrd=off  block_type=concat
      settings: block_version=10.1.3
  Concat3 : xbsIndex_r4/Concat  num_inputs=2  dbl_ovrd=off  block_type=concat
      settings: block_version=10.1.3
  Constant1 : xbsIndex_r4/Constant  arith_type=Unsigned  const=7  n_bits=3  bin_pt=0  explicit_period=on  period=1  equ=P=C  opselect=C  inp2=PCIN>>17  opr=+  inp1=P  carry=CIN  dbl_ovrd=off  block_type=constant
  Constant14 : xbsIndex_r4/Constant  arith_type=Unsigned  const=5  n_bits=16  bin_pt=0  explicit_period=on  period=1  equ=P=C  opselect=C  inp2=PCIN>>17  opr=+  inp1=P  carry=CIN  dbl_ovrd=off  block_type=constant
  Constant2 : xbsIndex_r4/Constant  arith_type=Unsigned  const=7  n_bits=3  bin_pt=0  explicit_period=on  period=1  equ=P=C  opselect=C  inp2=PCIN>>17  opr=+  inp1=P  carry=CIN  dbl_ovrd=off  block_type=constant
  Constant3 : xbsIndex_r4/Constant  arith_type=Unsigned  const=magic_id  n_bits=16  bin_pt=0  explicit_period=on  period=1  equ=P=C  opselect=C  inp2=PCIN>>17  opr=+  inp1=P  carry=CIN  dbl_ovrd=off  block_type=constant
  Constant4 : xbsIndex_r4/Constant  arith_type=Unsigned  const=ver_id  n_bits=16  bin_pt=0  explicit_period=on  period=1  equ=P=C  opselect=C  inp2=PCIN>>17  opr=+  inp1=P  carry=CIN  dbl_ovrd=off  block_type=constant
  Constant5 : xbsIndex_r4/Constant  arith_type=Unsigned  const=0  n_bits=16  bin_pt=0  explicit_period=on  period=1  equ=P=C  opselect=C  inp2=PCIN>>17  opr=+  inp1=P  carry=CIN  dbl_ovrd=off  block_type=constant
  Constant6 : xbsIndex_r4/Constant  arith_type=Unsigned  const=6  n_bits=16  bin_pt=0  explicit_period=on  period=1  equ=P=C  opselect=C  inp2=PCIN>>17  opr=+  inp1=P  carry=CIN  dbl_ovrd=off  block_type=constant
  Constant7 : xbsIndex_r4/Constant  arith_type=Unsigned  const=7-1  n_bits=3  bin_pt=0  explicit_period=on  period=1  equ=P=C  opselect=C  inp2=PCIN>>17  opr=+  inp1=P  carry=CIN  dbl_ovrd=off  block_type=constant
  Constant8 : xbsIndex_r4/Constant  arith_type=Unsigned  const=51  n_bits=16  bin_pt=0  explicit_period=on  period=1  equ=P=C  opselect=C  inp2=PCIN>>17  opr=+  inp1=P  carry=CIN  dbl_ovrd=off  block_type=constant
  Convert1 : xbsIndex_r4/Convert  arith_type=Unsigned  n_bits=24  bin_pt=0  quantization=Truncate  overflow=Wrap  latency=0  dbl_ovrd=off  pipeline=off  block_type=convert
      settings: block_version=10.1.3
  Convert2 : xbsIndex_r4/Convert  arith_type=Unsigned  n_bits=48  bin_pt=0  quantization=Truncate  overflow=Wrap  latency=0  dbl_ovrd=off  pipeline=off  block_type=convert
      settings: block_version=10.1.3
  Convert3 : xbsIndex_r4/Convert  arith_type=Unsigned  n_bits=24  bin_pt=0  quantization=Truncate  overflow=Wrap  latency=0  dbl_ovrd=off  pipeline=off  block_type=convert
      settings: block_version=10.1.3
  Counter1 : xbsIndex_r4/Counter  cnt_type=Free Running  cnt_to=1023  operation=Up  start_count=0  cnt_by_val=1  arith_type=Unsigned  n_bits=15  bin_pt=0  load_pin=off  rst=on  en=on  explicit_period=on  period=1  dbl_ovrd=off  use_behavioral_HDL=off  use_rpm=on  implementation=Fabric  block_type=counter
      settings: xl_area=[0, 0, 0, 0, 0, 0, 0]
  Counter2 : xbsIndex_r4/Counter  cnt_type=Free Running  cnt_to=1023  operation=Up  start_count=0  cnt_by_val=1  arith_type=Unsigned  n_bits=vector_bits+1  bin_pt=0  load_pin=off  rst=on  en=on  explicit_period=on  period=1  dbl_ovrd=off  use_behavioral_HDL=off  use_rpm=on  implementation=Fabric  block_type=counter
      settings: xl_area=[0, 0, 0, 0, 0, 0, 0]
  Counter3 : xbsIndex_r4/Counter  cnt_type=Free Running  cnt_to=1023  operation=Up  start_count=0  cnt_by_val=1  arith_type=Unsigned  n_bits=24  bin_pt=0  load_pin=off  rst=on  en=on  explicit_period=on  period=1  dbl_ovrd=off  use_behavioral_HDL=off  use_rpm=on  implementation=Fabric  block_type=counter
      settings: xl_area=[0, 0, 0, 0, 0, 0, 0]
  Gateway Out{1..7,14} (8 alike) : xbsIndex_r4/Gateway Out  hdl_port=on  timing_constraint=None  locs_specified=off  LOCs={}  block_type=gatewayout
      settings: infoedit="Gateway out block.  Converts Xilinx fixed point inputs into ouputs of type Simulink integer, double, or fixed point.<P><P>Hardware notes:  In hardware these blocks become top level output ports or are discarded, depending on how they are configured."  xl_area=[0, 0, 0, 0, 0, 0, 0]  block_version=10.1.3
  Inverter1 : xbsIndex_r4/Inverter  en=off  latency=0  dbl_ovrd=off  block_type=inv
      settings: xl_area=[0, 0, 0, 0, 0, 0, 0]
  Inverter2 : xbsIndex_r4/Inverter  en=off  latency=0  dbl_ovrd=off  block_type=inv
      settings: xl_area=[0, 0, 0, 0, 0, 0, 0]
  Inverter3 : xbsIndex_r4/Inverter  en=off  latency=0  dbl_ovrd=off  block_type=inv
      settings: xl_area=[0, 0, 0, 0, 0, 0, 0]
  Logical1 : xbsIndex_r4/Logical  logical_function=AND  inputs=2  en=off  latency=0  precision=Full  arith_type=Unsigned  n_bits=8  bin_pt=2  align_bp=on  dbl_ovrd=off  block_type=logical
      settings: xl_area=[0, 0, 0, 0, 0, 0, 0]
  Logical2 : xbsIndex_r4/Logical  logical_function=AND  inputs=2  en=off  latency=0  precision=Full  arith_type=Unsigned  n_bits=8  bin_pt=2  align_bp=on  dbl_ovrd=off  block_type=logical
      settings: xl_area=[0, 0, 0, 0, 0, 0, 0]
  Logical4 : xbsIndex_r4/Logical  logical_function=AND  inputs=2  en=off  latency=0  precision=Full  arith_type=Unsigned  n_bits=8  bin_pt=2  align_bp=on  dbl_ovrd=off  block_type=logical
      settings: xl_area=[0, 0, 0, 0, 0, 0, 0]
  Logical5 : xbsIndex_r4/Logical  logical_function=OR  inputs=2  en=off  latency=0  precision=Full  arith_type=Unsigned  n_bits=8  bin_pt=2  align_bp=on  dbl_ovrd=off  block_type=logical
      settings: xl_area=[0, 0, 0, 0, 0, 0, 0]
  Mult : xbsIndex_r4/Mult  precision=Full  arith_type="Signed  (2's comp)"  n_bits=16  bin_pt=14  quantization=Truncate  overflow=Wrap  en=off  latency=4  dbl_ovrd=off  use_behavioral_HDL=off  use_embedded=on  opt=Speed  optimum_pipeline=on  pipeline=on  use_rpm=on  placement_style=Triangular  block_type=mult
      settings: infoedit=Hardware notes: To use the internal pipeline stage of the dedicated multiplier you must select 'Pipeline for maximum performance'.  block_version=10.1.3
  Mux1 : xbsIndex_r4/Mux  inputs=8  en=off  latency=0  precision=Full  arith_type="Signed  (2's comp)"  n_bits=8  bin_pt=2  quantization=Truncate  overflow=Wrap  dbl_ovrd=off  block_type=mux
      settings: xl_area=[0, 0, 0, 0, 0, 0, 0]
  Mux2 : xbsIndex_r4/Mux  inputs=2  en=off  latency=0  precision=Full  arith_type="Signed  (2's comp)"  n_bits=8  bin_pt=2  quantization=Truncate  overflow=Wrap  dbl_ovrd=off  block_type=mux
      settings: xl_area=[0, 0, 0, 0, 0, 0, 0]
  Register : xbsIndex_r4/Register  init=0  rst=on  en=on  dbl_ovrd=off  block_type=register
  Relational1 : xbsIndex_r4/Relational  mode=a>=b  en=off  latency=0  dbl_ovrd=off  block_type=relational
      settings: xl_area=[0, 0, 0, 0, 0, 0, 0]  block_version=10.1.3
  Relational2 : xbsIndex_r4/Relational  mode=a<b  en=off  latency=0  dbl_ovrd=off  block_type=relational
      settings: xl_area=[0, 0, 0, 0, 0, 0, 0]  block_version=10.1.3
  lsb : xbsIndex_r4/Slice  nbits=3  boolean_output=off  mode=Lower Bit Location + Width  bit1=0  base1=MSB of Input  bit0=0  base0=LSB of Input  dbl_ovrd=off  block_type=slice
      settings: infoedit="Extracts a given range of bits from each input sample and presents it at the output.  The output type is ordinarily unsigned with binary point at zero, but can be Boolean when the slice is one bit wide.<P><P>Hardware notes: In hardware this block costs nothing."  block_version=10.1.3
  lsb1 : xbsIndex_r4/Slice  nbits=11  boolean_output=off  mode=Lower Bit Location + Width  bit1=0  base1=MSB of Input  bit0=3  base0=LSB of Input  dbl_ovrd=off  block_type=slice
      settings: infoedit="Extracts a given range of bits from each input sample and presents it at the output.  The output type is ordinarily unsigned with binary point at zero, but can be Boolean when the slice is one bit wide.<P><P>Hardware notes: In hardware this block costs nothing."  block_version=10.1.3
  lsb2 : xbsIndex_r4/Slice  nbits=14  boolean_output=off  mode=Lower Bit Location + Width  bit1=0  base1=MSB of Input  bit0=0  base0=LSB of Input  dbl_ovrd=off  block_type=slice
      settings: infoedit="Extracts a given range of bits from each input sample and presents it at the output.  The output type is ordinarily unsigned with binary point at zero, but can be Boolean when the slice is one bit wide.<P><P>Hardware notes: In hardware this block costs nothing."  block_version=10.1.3
  packetise_output : Scope  NumInputPorts=8
      settings: YMin=0~0~0~0~0~0~0~-5  YMax=1200~1~5~1~100~1~1~5
  posedge : casper_library/Misc/posedge  Tag=Rising Edge Detector  SystemSampleTime=-1
  data_out : Outport  OutDataType=sfix(16)  OutScaling=2^0
  valid_out : Outport  Port=2  OutDataType=sfix(16)  OutScaling=2^0
  dest_ip : Outport  Port=3  OutDataType=sfix(16)  OutScaling=2^0
  eof : Outport  Port=4  OutDataType=sfix(16)  OutScaling=2^0
  ack_out : Outport  Port=5  OutDataType=sfix(16)  OutScaling=2^0
  wires:
  [ack_output] -> Gateway Out2/1
  [writing_header] -> Gateway Out5/1
  [end_of_integration] -> Gateway Out14/1
  Gateway Out14/1 -> packetise_output/7
  [valid_input] -> Gateway Out4/1
  [start_new_packet] -> Gateway Out6/1
  [end_of_integration] -> Logical5/1
  Gateway Out6/1 -> packetise_output/6
  Gateway Out5/1 -> packetise_output/5
  Gateway Out2/1 -> packetise_output/4
  Gateway Out1/1 -> packetise_output/3
  Gateway Out4/1 -> packetise_output/2
  Gateway Out3/1 -> packetise_output/1
  ip_addr/1 -> dest_ip/1
  valid_in/1 -> [valid_input], Logical2/1
  Mux1/1 -> data_out/1, [data_out]
  Logical5/1 -> posedge/1
  Counter1/1 -> Relational2/1, lsb/1, Relational1/1
  [valid_input] -> Counter1/2
  [start_new_packet] -> Counter1/1
  Relational2/1 -> [writing_header], Mux2/1
  Constant1/1 -> Relational2/2
  Mux2/1 -> [output_sel]
  [output_sel] -> Mux1/1
  [output_sel] -> Gateway Out1/1
  [data_out] -> Gateway Out3/1
  Inverter1/1 -> ack_out/1, [ack_output]
  [writing_header] -> Inverter1/1
  Logical2/1 -> [end_of_integration]
  vector_complete/1 -> Logical2/2
  data_in/1 -> Assert6/1
  opt1/1 -> Assert/1
  Assert/1 -> [header_opt1]
  Assert1/1 -> [header_opt2]
  Assert2/1 -> [header_opt3]
  Assert3/1 -> [header_opt4]
  opt2/1 -> Assert1/1
  opt3/1 -> Assert2/1
  opt4/1 -> Assert3/1
  [header_opt1] -> Mux1/3
  Concat/1 -> Mux1/2
  Constant3/1 -> Concat/1
  Constant4/1 -> Concat/2
  Constant5/1 -> Concat/3
  Constant6/1 -> Concat/4
  [data_input] -> Mux1/9
  [header_opt2] -> Mux1/4
  [header_opt3] -> Mux1/5
  [header_opt4] -> Mux1/6
  Concat1/1 -> Mux1/7
  Assert6/1 -> [data_input]
  Constant2/1 -> Mux2/2
  lsb/1 -> Mux2/3
  Relational1/1 -> Register/1, Register/3, Inverter2/1
  Register/1 -> Logical5/2
  [valid_input] -> Logical1/2
  posedge/1 -> [start_new_packet]
  [start_new_packet] -> Logical4/1
  AddSub/1 -> Relational1/2
  pkt_len (bytes)/1 -> lsb2/1
  Constant7/1 -> AddSub/2
  lsb1/1 -> AddSub/1
  Inverter2/1 -> Logical1/1
  Logical1/1 -> Register/2
  [valid_input] -> valid_out/1
  Constant14/1 -> Concat3/1
  [vector_position] -> Convert2/1
  Concat3/1 -> Mux1/8
  Counter2/1 -> Mult/1
  [eof] -> Counter2/2
  [payload_len] -> Mult/2
  Mult/1 -> [vector_position]
  [end_of_integration] -> Counter2/1
  Gateway Out7/1 -> packetise_output/8
  [vector_position] -> Gateway Out7/1
  Convert2/1 -> Concat3/2
  Constant8/1 -> Concat1/1
  Convert1/1 -> Concat1/2
  [payload_len] -> Convert1/1
  lsb2/1 -> lsb1/1, [payload_len]
  Convert3/1 -> Concat1/3
  Counter3/1 -> Convert3/1
  [end_of_integration] -> Counter3/1
  [start_new_packet] -> Counter3/2
  Logical4/1 -> eof/1, [eof]
  Inverter3/1 -> Logical4/2
  [writing_header] -> Inverter3/1
